simulink model "productionLine2machines_heuristicPolicy"  (R2024b)
settings: Solver=VariableStepAuto  StartTime=0.0  StopTime=2000  RelTol=1e-3
model workspace (MAT data in the model file):
  bufferCapacity1 = 50
  bufferProcessedProducts = 50
undefined symbols (not defined in the file): m, n, T1, T2
settings Model: Creator=giopa  LastModifiedBy=giopa
settings DataIOCC: InspectSignalLogs=on

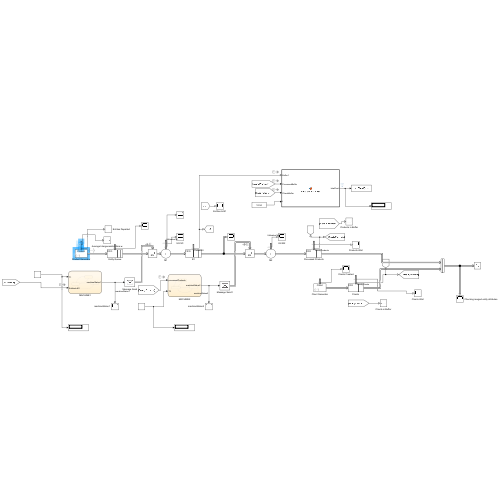
[thumbnail: Simulink's stored preview of the top-level diagram]
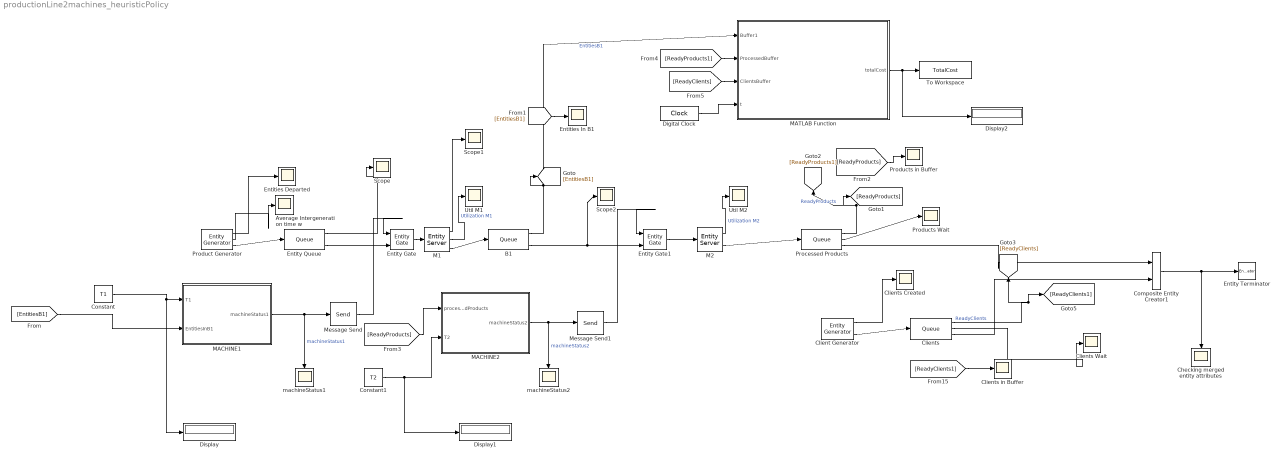
== system productionLine2machines_heuristicPolicy ==
  Average Intergeneration time w : Scope
  B1 : Queue  InputPortMessageModes=m  OutputPortMessageModes=n,m  Capacity=bufferCapacity1  NumberEntitiesInBlock=on
      settings: OutputPortMap=o1,o5
  Checking merged entity attributes : Scope
  Client Generator : EntityGenerator  OutputPortMessageModes=n,m  TimeSource=MATLAB action  IntergenerationTimeAction=|  GenerateEntityAtSimulationStart=off  GenerateAction=|  AttributeName=clientNumber  NumberEntitiesDeparted=on  EntityType=Structured  EntityTypeName=Client
      IntergenerationTimeAction=|
      | muI = 4.5;   % Mean intergeneration time 
      | dt = -muI * log(1 - rand());  % Exponential distribution
      GenerateAction=|
      | persistent clientNumber;
      | if isempty(clientNumber)
      |     clientNumber = 0; % Initialize the first client number
      | else
      |     clientNumber = clientNumber + 1; % Increment client number for each new entity
      | end
      | entity.clientNumber = clientNumber; % Assign the number to the entity's attribute
      settings: OutputPortMap=o0,o3
  "Clients " : Queue  InputPortMessageModes=m  OutputPortMessageModes=n,n,m  Capacity=50  NumberEntitiesInBlock=on  AverageWait=on
      settings: OutputPortMap=o1,o2,o5
  Clients Created : Scope
  Clients Wait : Scope
  Clients in Buffer : Scope
  Composite Entity Creator1 : CompositeEntityCreator  InputPortMessageModes=m,m  OutputPortMessageModes=m  EntityTypeName=Order  InputEntityName=Product|Client
      settings: InputPortMap=u0,u1
  Constant : Constant  Value=T1
  Constant1 : Constant  Value=T2
  Digital Clock : DigitalClock  SampleTime=0.1
  Display : Display
  Display1 : Display
  Display2 : Display
  Entities Departed : Scope
  Entities In B1 : Scope
  Entity Gate : EntityGate  InputPortMessageModes=m,m  OutputPortMessageModes=m  MatchingAttributeName=gateCheck  InitialValueOfMatchingAttribute=1  OpenGateAtSimulationStart=on
  Entity Gate1 : EntityGate  InputPortMessageModes=m,m  OutputPortMessageModes=m  MatchingAttributeName=machineStatus  InitialValueOfMatchingAttribute=1
  Entity Queue : Queue  InputPortMessageModes=m  OutputPortMessageModes=n,m  Capacity=500  NumberEntitiesInBlock=on
      settings: OutputPortMap=o1,o5
  Entity Terminator : EntityTerminator  InputPortMessageModes=m
  M1 : EntityServer  InputPortMessageModes=m  OutputPortMessageModes=n,n,m  Capacity=1  ServiceTimeSource=Attribute  ServiceTimeValue=1  ServiceTimeAttributeName=processingTime  NumberEntitiesInBlock=on  Utilization=on
      settings: OutputPortMap=o1,o5,o9
  M2 : EntityServer  InputPortMessageModes=m  OutputPortMessageModes=n,m  Capacity=1  ServiceTimeSource=Attribute  ServiceTimeValue=1  ServiceTimeAttributeName=processingTime  Utilization=on
      settings: OutputPortMap=o5,o9
  MACHINE1 : Stateflow chart  TreatAsAtomicUnit=on
  MACHINE2 : Stateflow chart  TreatAsAtomicUnit=on
  MATLAB Function : MATLAB Function  TreatAsAtomicUnit=on
  Message Send : Send  OutputPortMessageModes=m
  Message Send1 : Send  OutputPortMessageModes=m
  Processed Products : Queue  InputPortMessageModes=m  OutputPortMessageModes=n,n,m  Capacity=bufferProcessedProducts  NumberEntitiesInBlock=on  AverageWait=on
      settings: OutputPortMap=o1,o2,o5
  Product Generator : EntityGenerator  OutputPortMessageModes=n,n,m  Period=2  IntergenerationTimeAction=|  GenerateAction=|  ExitAction=|  AttributeName=processingTime|productNumber|entryTime  AttributeInitialValue=2|1|1  NumberEntitiesDeparted=on  AverageIntergenerationTime=on  EntityType=Structured  EntityTypeName=Product
      IntergenerationTimeAction=|
      | muI = 2;   % Mean intergeneration time 
      | dt = -muI * log(1 - rand());  % Exponential distribution
      GenerateAction=|
      | persistent rngInit;
      | if isempty(rngInit)
      |     seed = 12345;
      |     rng(seed);
      |     rngInit = true;
      | end
      | % Pattern: Exponential distribution
      | 
      | mu = 2;
      | entity.processingTime = -mu * log(1 - rand());
      | 
      | %assign productNumber aatribute to every entity
      | persistent productNumber
      | if isempty(productNumber)
      |     productNumber = 0;  
      | end
      | 
      | % Assign productNumber attribute
      | entity.productNumber = productNumber + 1; % Increment and assign the product number
      | productNumber = productNumber + 1;        % Update the product number for the next product
      ExitAction=|
      | persistent productNumber;
      | if isempty(productNumber)
      |     productNumber = 1; % Initialize the first client number
      | else
      |     productNumber = productNumber + 1; % Increment client number for each new entity
      | end
      | entity.productNumber = productNumber; % Assign the number to the entity's attribute
      settings: OutputPortMap=o0,o2,o3
  Products Wait : Scope
  Products in Buffer : Scope
  Scope : Scope
  Scope1 : Scope
  Scope2 : Scope
  To Workspace : ToWorkspace  VariableName=TotalCost  SaveFormat=Timeseries  SampleTime=-1
      settings: Save2DSignal=2-D array (concatenate along first dimension)
  Util M1 : Scope
  Util M2 : Scope
  machineStatus1 : Scope
  machineStatus2 : Scope
  wires:
  B1/2 -> Scope2/1, Entity Gate1/2
  M2/2 -> Processed Products/1
  Message Send1/1 -> Entity Gate1/1
  M1/2 -> Util M1/1  "Utilization M1"
  M2/1 -> Util M2/1  "Utilization M2"
  Entity Gate/1 -> M1/1
  "Clients "/2 -> Clients Wait/1
  [ReadyClients1] -> Clients in Buffer/1
  "Clients "/1 -> [ReadyClients1], [ReadyClients]  "ReadyClients"
  M1/3 -> B1/1
  Processed Products/3 -> Composite Entity Creator1/1
  Message Send/1 -> Entity Gate/1
  Processed Products/2 -> Products Wait/1
  Client Generator/1 -> Clients Created/1
  Product Generator/2 -> Average Intergeneration time w/1
  MACHINE1/1(machineStatus1) -> machineStatus1/1, Message Send/1  "machineStatus1"
  Entity Gate1/1 -> M2/1
  Composite Entity Creator1/1 -> Entity Terminator/1, Checking merged entity attributes/1
  MACHINE2/1(machineStatus2) -> Message Send1/1, machineStatus2/1  "machineStatus2"
  "Clients "/3 -> Composite Entity Creator1/2
  Product Generator/1 -> Entities Departed/1
  Client Generator/2 -> "Clients "/1
  B1/1 -> MATLAB Function/1(Buffer1), [EntitiesB1]  "EntitiesB1"
  [EntitiesB1] -> MACHINE1/2(EntitiesInB1)
  [EntitiesB1] -> Entities In B1/1
  Constant/1 -> Display/1, MACHINE1/1(T1)
  Processed Products/1 -> [ReadyProducts1], [ReadyProducts]  "ReadyProducts"
  [ReadyProducts] -> Products in Buffer/1
  [ReadyProducts] -> MACHINE2/1(processedProducts)
  Constant1/1 -> MACHINE2/2(T2), Display1/1
  MATLAB Function/1(totalCost) -> Display2/1, To Workspace/1
  Digital Clock/1 -> MATLAB Function/4(t)
  [ReadyProducts1] -> MATLAB Function/2(ProcessedBuffer)
  [ReadyClients] -> MATLAB Function/3(ClientsBuffer)
  Product Generator/3 -> Entity Queue/1
  Entity Queue/2 -> Entity Gate/2
  Entity Queue/1 -> Scope/1
  M1/1 -> Scope1/1

== stateflow chart productionLine2machines_heuristicPolicy/MACHINE2 ==
  state Failed
    entry:
    machineStatus2 = 0;
    repairTime2 = -meanRepairTime2 * log(1 - rand());
  state Idle
    entry:
    machineStatus2 = -1;
  state Working
    entry:
    machineStatus2 = 1;
    timeToFailure2 = -meanFailureTime2 * log(1 - rand());
  Working -> Failed [order 1] : [after(timeToFailure2, sec)]
  Failed -> Working : [after(repairTime2, sec)]
  (default) -> Working
  Idle -> Working : [processedProducts < (T2-1)]
  Working -> Idle [order 2] : [processedProducts >= T2]
  data: meanRepairTime2 constant double =5; meanFailureTime2 constant double =50; machineStatus2 output; repairTime2 local; timeToFailure2 local; processedProducts input; T2 input

== matlab function productionLine2machines_heuristicPolicy/MATLAB Function ==
  data: Buffer1 input; totalCost output; ProcessedBuffer input; ClientsBuffer input; t input
function totalCost = calculateTotalCost(Buffer1, ProcessedBuffer, ClientsBuffer, t)
    % Cost weights (as provided)
    w1 = 0.5;    % Cost for Buffer1 (between machines)
    w2 = 1;      % Cost for Processed Products Buffer
    w3 = 1.3;    % Cost for Clients Buffer

    % Persistent variable for last time
    persistent lastTime
    if isempty(lastTime)
        lastTime = t;
        totalCost = 0; % Initialize cost to zero
        return;
    end

    % Calculate dt from the difference between the current and last time
    dt = t - lastTime;
    lastTime = t;

    % Cost calculation for the current time step
    totalCost = (Buffer1*w1 + ProcessedBuffer*w2 + ClientsBuffer*w3)*dt;
end

== stateflow chart productionLine2machines_heuristicPolicy/MACHINE1 ==
  state Failed
    entry:
    machineStatus1 = 0;
    repairTime1 = -meanRepairTime1 * log(1 - rand());
  state Idle
    entry:
    machineStatus1 = -1;
  state Working
    entry:
    machineStatus1 = 1;
    timeToFailure1 = -meanFailureTime1 * log(1 - rand());
  Working -> Failed [order 1] : [after(timeToFailure1, sec)]
  Failed -> Working : [after(repairTime1, sec)]
  (default) -> Working
  Idle -> Working : [EntitiesInB1 <=(T1-1)]
  Working -> Idle [order 2] : [EntitiesInB1 >= T1]
  data: meanRepairTime1 constant double =5; meanFailureTime1 constant double =50; machineStatus1 output; repairTime1 local; timeToFailure1 local; T1 input; EntitiesInB1 input
